simulink model "CircuitRealization"  (R2020b)
settings: Solver=VariableStepAuto  StartTime=0.0  StopTime=10.0  RelTol=1e-3
settings Model: Creator=baner  LastModifiedBy=baner

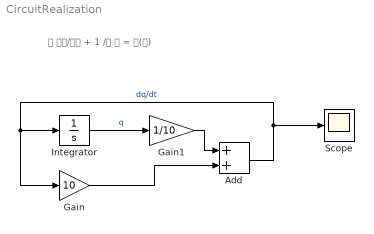
== system CircuitRealization ==
  note: 𝑅 𝑑𝑄/𝑑𝑡 + 1 /𝐶 𝑄 = 𝐸(𝑡)
  Add : Sum
  Gain : Gain  Gain=10
  Gain1 : Gain  Gain=1/10
  Integrator : Integrator
  Scope : Scope
  wires:
  Integrator/1 -> Gain1/1  "q"
  Add/1 -> Gain/1, Integrator/1, Scope/1  "dq/dt"
  Gain1/1 -> Add/1
  Gain/1 -> Add/2
